simulink model "rmc_simulation"  (R2022b)
settings: Solver=ode45  StartTime=0.0  StopTime=50  FixedStep=0.01  RelTol=1e-3
settings Model: SimulationMode=accelerator  Creator=Adith JB  LastModifiedBy=Rohit
settings SolverCC: AlgebraicLoopSolver=TrustRegion
settings DataIOCC: LimitDataPoints=on  SaveFormat=Array  SignalLoggingSaveFormat=ModelDataLogs  ReturnWorkspaceOutputs=off
settings OptimizationCC: BlockReduction=off  BooleanDataType=off  ExpressionDepthLimit=2147483647  LifeSpan=inf
settings DebuggingCC: SaveWithParameterizedLinksMsg=none  UnderspecifiedInitializationDetection=Classic  MergeDetectMultiDrivingBlocksExec=none  SignalResolutionControl=TryResolveAllWithWarning  MultiTaskDSMMsg=warning  MultiTaskCondExecSysMsg=none  UnconnectedInputMsg=warning  UnconnectedOutputMsg=warning  UnconnectedLineMsg=warning  StateNameClashWarn=warning  SFUnexpectedBacktrackingDiag=warning  SFNoUnconditionalDefaultTransitionDiag=warning  SFExecutionAtInitializationDiag=none  SFMachineParentedDataDiag=warning  ArithmeticOperatorsInVariantConditions=warning
settings HardwareCC: ProdBitPerPointer=32  ProdBitPerSizeT=32  ProdBitPerPtrDiffT=32  ProdLargestAtomicFloat=None  ProdIntDivRoundTo=Undefined  ProdEndianess=Unspecified  ProdWordSize=32  ProdHWDeviceType=32-bit Generic  TargetUnknown=on
settings ModelReferenceCC: PropagateSignalLabelsOutOfModel=off
settings SFSimCC: SimUseLocalCustomCode=off  CustomCodeUndefinedFunction=UseInterfaceOnly
settings RTWCC: RTWUseLocalCustomCode=off
settings CodeAppCC: StateflowObjectComments=on
settings GRTTargetCC: TargetLangStandard=C89/C90 (ANSI)
settings ConfigComp: CovMetricSettings=dw  CovSaveCumulativeToWorkspaceVar=on  CovSaveSingleToWorkspaceVar=on  CovExternalEMLEnable=off

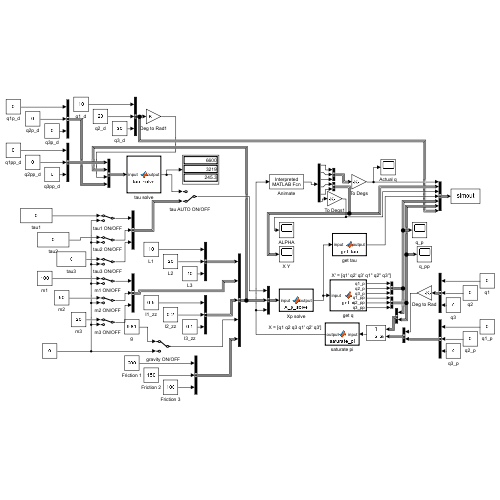
[thumbnail: Simulink's stored preview of the top-level diagram]
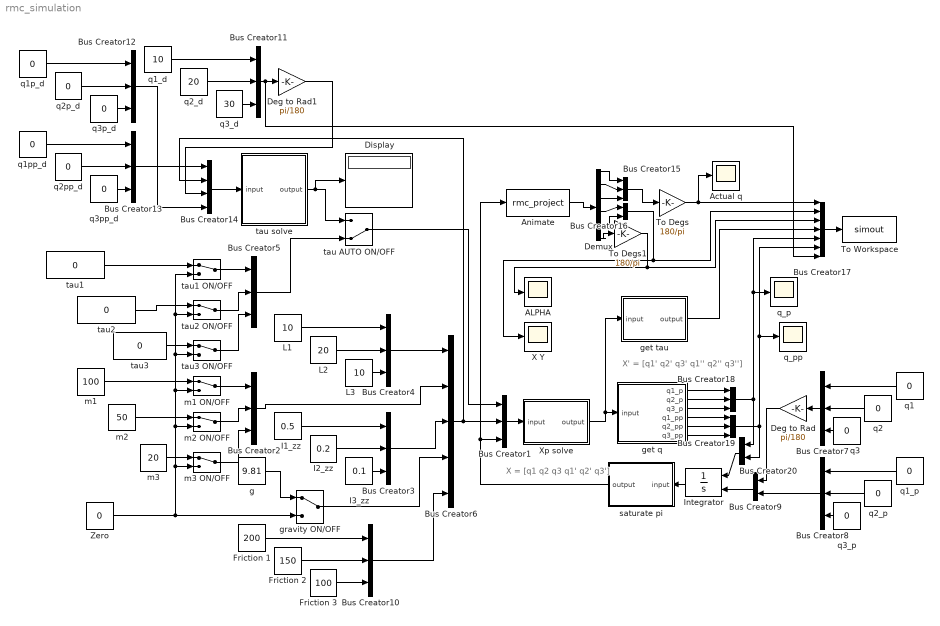
== system rmc_simulation ==
  note: X = [q1 q2 q3 q1' q2' q3']
  note: X' = [q1' q2' q3' q1'' q2'' q3'']
  ALPHA : Scope
  Actual q : Scope
  Animate : MATLABFcn  MATLABFcn=rmc_project  OutputDimensions=6  OutputSignalType=real
  Bus Creator{1..5,7..8,10..13,15,18..19} (14 alike) : BusCreator  Inputs=3
  Bus Creator14 : BusCreator  Inputs=4
  Bus Creator16 : BusCreator  Inputs=2
  Bus Creator17 : BusCreator  Inputs=7
  Bus Creator20 : BusCreator  Inputs=2
  Bus Creator6 : BusCreator  Inputs=5
  Bus Creator9 : BusCreator  Inputs=2
  Deg to Rad : Gain  Gain=pi/180
  Deg to Rad1 : Gain  Gain=pi/180
  Demux : Demux  Outputs=6
  Display : Display
  Friction 1 : Constant  Value=200
  Friction 2 : Constant  Value=150
  Friction 3 : Constant  Value=100
  I1_zz : Constant  Value=0.5
  I2_zz : Constant  Value=0.2
  I3_zz : Constant  Value=0.1
  Integrator : Integrator  InitialConditionSource=external
  L1 : Constant  Value=10
  L2 : Constant  Value=20
  L3 : Constant  Value=10
  To Degs : Gain  Gain=180/pi
  To Degs1 : Gain  Gain=180/pi
  To Workspace : ToWorkspace  VariableName=simout  SaveFormat=Structure With Time  SampleTime=-1
  X Y : Scope
  Xp solve : MATLAB Function  TreatAsAtomicUnit=on
  Zero : Constant  Value=0
  g : Constant  Value=9.81
  get q : MATLAB Function  TreatAsAtomicUnit=on
  get tau : MATLAB Function  TreatAsAtomicUnit=on
  gravity ON/OFF : ManualSwitch
  m1 : Constant  Value=100
  m1 ON/OFF : ManualSwitch
  m2 : Constant  Value=50
  m2 ON/OFF : ManualSwitch
  m3 : Constant  Value=20
  m3 ON/OFF : ManualSwitch
  q1 : Constant  Value=0
  q1_d : Constant  Value=10
  q1_p : Constant  Value=0
  q1p_d : Constant  Value=0
  q1pp_d : Constant  Value=0
  q2 : Constant  Value=0
  q2_d : Constant  Value=20
  q2_p : Constant  Value=0
  q2p_d : Constant  Value=0
  q2pp_d : Constant  Value=0
  q3 : Constant  Value=0
  q3_d : Constant  Value=30
  q3_p : Constant  Value=0
  q3p_d : Constant  Value=0
  q3pp_d : Constant  Value=0
  q_p : Scope
  q_pp : Scope
  saturate pi : MATLAB Function  TreatAsAtomicUnit=on
  tau AUTO ON/OFF : ManualSwitch  CurrentSetting=0
  tau solve : MATLAB Function  TreatAsAtomicUnit=on
  tau1 : Constant  Value=0
  tau1 ON/OFF : ManualSwitch
  tau2 : Constant  Value=0
  tau2 ON/OFF : ManualSwitch
  tau3 : Constant  Value=0
  tau3 ON/OFF : ManualSwitch
  wires:
  I1_zz/1 -> Bus Creator3/1
  I2_zz/1 -> Bus Creator3/2
  I3_zz/1 -> Bus Creator3/3
  L1/1 -> Bus Creator4/1
  L2/1 -> Bus Creator4/2
  L3/1 -> Bus Creator4/3
  Bus Creator4/1 -> Bus Creator6/1
  Bus Creator2/1 -> Bus Creator6/2
  Bus Creator3/1 -> Bus Creator6/3
  g/1 -> gravity ON/OFF/1
  gravity ON/OFF/1 -> Bus Creator6/4
  Bus Creator1/1 -> Xp solve/1(input)
  Bus Creator6/1 -> Bus Creator14/2, Bus Creator1/2
  To Degs/1 -> Bus Creator17/1, Actual q/1
  q1/1 -> Bus Creator7/1
  q2/1 -> Bus Creator7/2
  q3/1 -> Bus Creator7/3
  q1_p/1 -> Bus Creator8/1
  q2_p/1 -> Bus Creator8/2
  q3_p/1 -> Bus Creator8/3
  Bus Creator8/1 -> Bus Creator9/2
  Bus Creator7/1 -> Deg to Rad/1
  Deg to Rad/1 -> Bus Creator9/1
  Bus Creator9/1 -> Integrator/2
  m1/1 -> m1 ON/OFF/1
  m3 ON/OFF/1 -> Bus Creator2/3
  m3/1 -> m3 ON/OFF/1
  m1 ON/OFF/1 -> Bus Creator2/1
  m2 ON/OFF/1 -> Bus Creator2/2
  m2/1 -> m2 ON/OFF/1
  Integrator/1 -> saturate pi/1(input)
  Friction 3/1 -> Bus Creator10/3
  Friction 2/1 -> Bus Creator10/2
  Friction 1/1 -> Bus Creator10/1
  Bus Creator10/1 -> Bus Creator6/5
  tau1/1 -> tau1 ON/OFF/1
  tau2/1 -> tau2 ON/OFF/1
  Zero/1 -> gravity ON/OFF/2, tau1 ON/OFF/2, tau2 ON/OFF/2, tau3 ON/OFF/2, m1 ON/OFF/2, m2 ON/OFF/2, m3 ON/OFF/2
  tau3/1 -> tau3 ON/OFF/1
  tau3 ON/OFF/1 -> Bus Creator5/3
  tau2 ON/OFF/1 -> Bus Creator5/2
  tau1 ON/OFF/1 -> Bus Creator5/1
  tau solve/1(output) -> Display/1, tau AUTO ON/OFF/1
  Bus Creator5/1 -> tau AUTO ON/OFF/2
  tau AUTO ON/OFF/1 -> Bus Creator1/1
  q1_d/1 -> Bus Creator11/1
  q2_d/1 -> Bus Creator11/2
  q3_d/1 -> Bus Creator11/3
  q1p_d/1 -> Bus Creator12/1
  q2p_d/1 -> Bus Creator12/2
  q3p_d/1 -> Bus Creator12/3
  q1pp_d/1 -> Bus Creator13/1
  q2pp_d/1 -> Bus Creator13/2
  q3pp_d/1 -> Bus Creator13/3
  Bus Creator13/1 -> Bus Creator14/1
  Bus Creator11/1 -> Bus Creator17/7, Deg to Rad1/1
  Deg to Rad1/1 -> Bus Creator14/3
  Bus Creator12/1 -> Bus Creator14/4
  Bus Creator14/1 -> tau solve/1(input)
  saturate pi/1(output) -> Animate/1, Bus Creator1/3
  get tau/1(output) -> Bus Creator17/4
  Xp solve/1(output) -> get tau/1(input), get q/1(input)
  Animate/1 -> Demux/1
  Demux/1 -> Bus Creator15/1
  Demux/2 -> Bus Creator15/2
  Demux/3 -> Bus Creator15/3
  Bus Creator15/1 -> To Degs/1
  Bus Creator17/1 -> To Workspace/1
  get q/1(q1_p) -> Bus Creator18/1
  get q/2(q2_p) -> Bus Creator18/2
  get q/3(q3_p) -> Bus Creator18/3
  get q/4(q1_pp) -> Bus Creator19/1
  get q/5(q2_pp) -> Bus Creator19/2
  get q/6(q3_pp) -> Bus Creator19/3
  Bus Creator19/1 -> Bus Creator17/6, q_pp/1, Bus Creator20/2
  Bus Creator20/1 -> Integrator/1
  Bus Creator18/1 -> Bus Creator20/1, Bus Creator17/5, q_p/1
  Demux/4 -> Bus Creator16/1
  Demux/5 -> Bus Creator16/2
  Bus Creator16/1 -> X Y/1, Bus Creator17/2
  Demux/6 -> To Degs1/1
  To Degs1/1 -> Bus Creator17/3, ALPHA/1

== matlab function rmc_simulation/Xp solve ==
  data: input input; output output
function output  = X_p_solve(input)
    tau1 = input(1);
    tau2 = input(2);
    tau3 = input(3);
    L1 = input(4);
    L2 = input(5);
    L3 = input(6);
    m1 = input(7);
    m2 = input(8);
    m3 = input(9);
    I1_zz = input(10);
    I2_zz = input(11);
    I3_zz = input(12);
    g = input(13);
    D1 = input(14);
    D2 = input(15);
    D3 = input(16);
    q1 = input(17);
    q2 = input(18);
    q3 = input(19);
    q1_p = input(20);
    q2_p = input(21);
    q3_p = input(22);
    q1 = atan2(sin(q1),cos(q1));
    q2 = atan2(sin(q2),cos(q2));
    q3 = atan2(sin(q3),cos(q3));
    q1_pp = (2*(32*I2_zz*I3_zz*tau1 - 32*I2_zz*I3_zz*tau2 + 8*I3_zz*L2^2*m2*tau1 + 8*I2_zz*L3^2*m3*tau1 - 8*I3_zz*L2^2*m2*tau2 + 32*I3_zz*L2^2*m3*tau1 - 8*I2_zz*L3^2*m3*tau2 - 32*I3_zz*L2^2*m3*tau2 - 32*D1*I2_zz*I3_zz*q1_p + 32*D2*I2_zz*I3_zz*q2_p + 4*L2^2*L3^2*m3^2*tau1 - 4*L2^2*L3^2*m3^2*tau2 + 2*L2^2*L3^2*m2*m3*tau1 - 2*L2^2*L3^2*m2*m3*tau2 - 4*L2^2*L3^2*m3^2*tau1*cos(2*q3) + 4*L2^2*L3^2*m3^2*tau2*cos(2*q3) - 4*D1*L2^2*L3^2*m3^2*q1_p + 4*D2*L2^2*L3^2*m3^2*q2_p - 8*D1*I3_zz*L2^2*m2*q1_p - 8*D1*I2_zz*L3^2*m3*q1_p - 32*D1*I3_zz*L2^2*m3*q1_p + 8*D2*I3_zz*L2^2*m2*q2_p + 8*D2*I2_zz*L3^2*m3*q2_p + 32*D2*I3_zz*L2^2*m3*q2_p - 1120*I2_zz*I3_zz*L1*g*cos(q1) - 85*L1*L2^2*L3^2*g*m3^2*cos(q1) - 15*L1*L2^2*L3^2*g*m3^2*cos(q1 + 2*q2 + 2*q3) + 4*I2_zz*L1^2*L3^2*m3^2*q1_p^2*sin(2*q2 + 2*q3) + 4*I3_zz*L1*L2^3*m2^2*q1_p^2*sin(q2) + 4*I3_zz*L1*L2^3*m2^2*q2_p^2*sin(q2) + 32*I3_zz*L1*L2^3*m3^2*q1_p^2*sin(q2) + 32*I3_zz*L1*L2^3*m3^2*q2_p^2*sin(q2) + 15*L1*L2^2*L3^2*g*m3^2*cos(q1 + 2*q2) + 35*L1*L2^2*L3^2*g*m3^2*cos(q1 - 2*q3) + 50*L1*L2^2*L3^2*g*m3^2*cos(q1 + 2*q3) - 2*D1*L2^2*L3^2*m2*m3*q1_p + 2*D2*L2^2*L3^2*m2*m3*q2_p - 140*I3_zz*L1*L2^2*g*m2*cos(q1) - 240*I2_zz*L1*L3^2*g*m3*cos(q1) - 840*I3_zz*L1*L2^2*g*m3*cos(q1) + 40*I2_zz*L1*L3^2*g*m3*cos(q1 + 2*q2 + 2*q3) + 4*D1*L2^2*L3^2*m3^2*q1_p*cos(2*q3) - 4*D2*L2^2*L3^2*m3^2*q2_p*cos(2*q3) + 140*I3_zz*L1*L2^2*g*m2*cos(q1 + 2*q2) + 280*I3_zz*L1*L2^2*g*m3*cos(q1 + 2*q2) - 8*L1*L2^2*L3*m3^2*tau3*cos(q2 + q3) - 4*L1*L2*L3^2*m3^2*tau2*cos(q2) + 4*L1*L2*L3^2*m3^2*tau3*cos(q2) - 16*I2_zz*L1*L3*m3*tau3*cos(q2 + q3) + 4*I3_zz*L1^2*L2^2*m2^2*q1_p^2*sin(2*q2) + 16*I3_zz*L1^2*L2^2*m3^2*q1_p^2*sin(2*q2) + 4*L1*L2*L3^2*m3^2*tau2*cos(q2 + 2*q3) + 8*L1*L2^2*L3*m3^2*tau3*cos(q2 - q3) - 4*L1*L2*L3^2*m3^2*tau3*cos(q2 + 2*q3) + 4*I2_zz*L1*L3^3*m3^2*q1_p^2*sin(q2 + q3) + 4*I2_zz*L1*L3^3*m3^2*q2_p^2*sin(q2 + q3) + 4*I2_zz*L1*L3^3*m3^2*q3_p^2*sin(q2 + q3) - 16*I3_zz*L1*L2*m2*tau2*cos(q2) + 16*I3_zz*L1*L2*m2*tau3*cos(q2) - 32*I3_zz*L1*L2*m3*tau2*cos(q2) + 32*I3_zz*L1*L2*m3*tau3*cos(q2) + 8*I2_zz*L1*L3^3*m3^2*q1_p*q2_p*sin(q2 + q3) + 8*I2_zz*L1*L3^3*m3^2*q1_p*q3_p*sin(q2 + q3) + 8*I2_zz*L1*L3^3*m3^2*q2_p*q3_p*sin(q2 + q3) + 16*D3*I2_zz*L1*L3*m3*q3_p*cos(q2 + q3) - 35*L1*L2^2*L3^2*g*m2*m3*cos(q1) + L1*L2^2*L3^3*m2*m3^2*q1_p^2*sin(q2 - q3) + L1*L2^2*L3^3*m2*m3^2*q2_p^2*sin(q2 - q3) - L1*L2^3*L3^2*m2*m3^2*q1_p^2*sin(q2 + 2*q3) + L1*L2^2*L3^3*m2*m3^2*q3_p^2*sin(q2 - q3) - L1*L2^3*L3^2*m2*m3^2*q2_p^2*sin(q2 + 2*q3) - 4*D2*L1*L2*L3^2*m3^2*q2_p*cos(q2 + 2*q3) - 8*D3*L1*L2^2*L3*m3^2*q3_p*cos(q2 - q3) + 4*D3*L1*L2*L3^2*m3^2*q3_p*cos(q2 + 2*q3) + 24*I3_zz*L1*L2^3*m2*m3*q1_p^2*sin(q2) + 24*I3_zz*L1*L2^3*m2*m3*q2_p^2*sin(q2) + 8*I3_zz*L1*L2^3*m2^2*q1_p*q2_p*sin(q2) + 64*I3_zz*L1*L2^3*m3^2*q1_p*q2_p*sin(q2) + 16*D2*I3_zz*L1*L2*m2*q2_p*cos(q2) + 32*D2*I3_zz*L1*L2*m3*q2_p*cos(q2) - 16*D3*I3_zz*L1*L2*m2*q3_p*cos(q2) - 32*D3*I3_zz*L1*L2*m3*q3_p*cos(q2) + 8*I3_zz*L1*L2^2*L3*m3^2*q1_p^2*sin(q2 + q3) + 8*I3_zz*L1*L2^2*L3*m3^2*q2_p^2*sin(q2 + q3) + 8*I3_zz*L1*L2^2*L3*m3^2*q3_p^2*sin(q2 + q3) + 25*L1*L2^2*L3^2*g*m2*m3*cos(q1 + 2*q2) - 10*L1*L2^2*L3^2*g*m2*m3*cos(q1 + 2*q3) + 4*I2_zz*L1*L2*L3^2*m3^2*q1_p^2*sin(q2) + 4*I2_zz*L1*L2*L3^2*m3^2*q2_p^2*sin(q2) + 16*I2_zz*I3_zz*L1*L3*m3*q1_p^2*sin(q2 + q3) + 16*I2_zz*I3_zz*L1*L3*m3*q2_p^2*sin(q2 + q3) + 16*I2_zz*I3_zz*L1*L3*m3*q3_p^2*sin(q2 + q3) + 4*I2_zz*L1*L2*L3^2*m3^2*q1_p^2*sin(q2 + 2*q3) + 8*I3_zz*L1*L2^2*L3*m3^2*q1_p^2*sin(q2 - q3) + 4*I2_zz*L1*L2*L3^2*m3^2*q2_p^2*sin(q2 + 2*q3) + 8*I3_zz*L1*L2^2*L3*m3^2*q2_p^2*sin(q2 - q3) + 8*I3_zz*L1*L2^2*L3*m3^2*q3_p^2*sin(q2 - q3) + 16*I2_zz*I3_zz*L1*L2*m2*q1_p^2*sin(q2) + 16*I2_zz*I3_zz*L1*L2*m2*q2_p^2*sin(q2) + 32*I2_zz*I3_zz*L1*L2*m3*q1_p^2*sin(q2) + 32*I2_zz*I3_zz*L1*L2*m3*q2_p^2*sin(q2) + 2*L1^2*L2^2*L3^2*m2*m3^2*q1_p^2*sin(2*q2) + L1^2*L2^2*L3^2*m2^2*m3*q1_p^2*sin(2*q2) - 4*L1*L2*L3^2*m2*m3*tau2*cos(q2) + 4*L1*L2*L3^2*m2*m3*tau3*cos(q2) + 8*D3*L1*L2^2*L3*m3^2*q3_p*cos(q2 + q3) - L1^2*L2^2*L3^2*m2*m3^2*q1_p^2*sin(2*q2 + 2*q3) + 16*I3_zz*L1^2*L2^2*m2*m3*q1_p^2*sin(2*q2) + 3*L1*L2^3*L3^2*m2*m3^2*q1_p^2*sin(q2) + L1*L2^3*L3^2*m2^2*m3*q1_p^2*sin(q2) + 3*L1*L2^3*L3^2*m2*m3^2*q2_p^2*sin(q2) + L1*L2^3*L3^2*m2^2*m3*q2_p^2*sin(q2) + 4*L1*L2^2*L3*m2*m3*tau3*cos(q2 - q3) + 4*D2*L1*L2*L3^2*m3^2*q2_p*cos(q2) - 4*D3*L1*L2*L3^2*m3^2*q3_p*cos(q2) + 6*L1*L2^3*L3^2*m2*m3^2*q1_p*q2_p*sin(q2) + 2*L1*L2^3*L3^2*m2^2*m3*q1_p*q2_p*sin(q2) + 4*D2*L1*L2*L3^2*m2*m3*q2_p*cos(q2) - 4*D3*L1*L2*L3^2*m2*m3*q3_p*cos(q2) + 2*L1*L2^2*L3^3*m2*m3^2*q1_p*q2_p*sin(q2 - q3) + 2*L1*L2^2*L3^3*m2*m3^2*q1_p*q3_p*sin(q2 - q3) - 2*L1*L2^3*L3^2*m2*m3^2*q1_p*q2_p*sin(q2 + 2*q3) + 2*L1*L2^2*L3^3*m2*m3^2*q2_p*q3_p*sin(q2 - q3) - 4*D3*L1*L2^2*L3*m2*m3*q3_p*cos(q2 - q3) + 48*I3_zz*L1*L2^3*m2*m3*q1_p*q2_p*sin(q2) + 16*I3_zz*L1*L2^2*L3*m3^2*q1_p*q2_p*sin(q2 + q3) + 16*I3_zz*L1*L2^2*L3*m3^2*q1_p*q3_p*sin(q2 + q3) + 16*I3_zz*L1*L2^2*L3*m3^2*q2_p*q3_p*sin(q2 + q3) + 4*I2_zz*L1*L2*L3^2*m2*m3*q1_p^2*sin(q2) + 4*I2_zz*L1*L2*L3^2*m2*m3*q2_p^2*sin(q2) + 8*I2_zz*L1*L2*L3^2*m3^2*q1_p*q2_p*sin(q2) + 32*I2_zz*I3_zz*L1*L3*m3*q1_p*q2_p*sin(q2 + q3) + 32*I2_zz*I3_zz*L1*L3*m3*q1_p*q3_p*sin(q2 + q3) + 32*I2_zz*I3_zz*L1*L3*m3*q2_p*q3_p*sin(q2 + q3) + 4*I3_zz*L1*L2^2*L3*m2*m3*q1_p^2*sin(q2 - q3) + 4*I3_zz*L1*L2^2*L3*m2*m3*q2_p^2*sin(q2 - q3) + 4*I3_zz*L1*L2^2*L3*m2*m3*q3_p^2*sin(q2 - q3) + 8*I2_zz*L1*L2*L3^2*m3^2*q1_p*q2_p*sin(q2 + 2*q3) + 16*I3_zz*L1*L2^2*L3*m3^2*q1_p*q2_p*sin(q2 - q3) + 16*I3_zz*L1*L2^2*L3*m3^2*q1_p*q3_p*sin(q2 - q3) + 16*I3_zz*L1*L2^2*L3*m3^2*q2_p*q3_p*sin(q2 - q3) + 32*I2_zz*I3_zz*L1*L2*m2*q1_p*q2_p*sin(q2) + 64*I2_zz*I3_zz*L1*L2*m3*q1_p*q2_p*sin(q2) + 8*I2_zz*L1*L2*L3^2*m2*m3*q1_p*q2_p*sin(q2) + 8*I3_zz*L1*L2^2*L3*m2*m3*q1_p*q2_p*sin(q2 - q3) + 8*I3_zz*L1*L2^2*L3*m2*m3*q1_p*q3_p*sin(q2 - q3) + 8*I3_zz*L1*L2^2*L3*m2*m3*q2_p*q3_p*sin(q2 - q3)))/(64*I1_zz*I2_zz*I3_zz + 16*I2_zz*I3_zz*L1^2*m1 + 16*I1_zz*I3_zz*L2^2*m2 + 64*I2_zz*I3_zz*L1^2*m2 + 16*I1_zz*I2_zz*L3^2*m3 + 64*I1_zz*I3_zz*L2^2*m3 + 64*I2_zz*I3_zz*L1^2*m3 + 8*I3_zz*L1^2*L2^2*m2^2 + 8*I1_zz*L2^2*L3^2*m3^2 + 8*I2_zz*L1^2*L3^2*m3^2 + 32*I3_zz*L1^2*L2^2*m3^2 - 8*I2_zz*L1^2*L3^2*m3^2*cos(2*q2 + 2*q3) + 2*L1^2*L2^2*L3^2*m1*m3^2 + 6*L1^2*L2^2*L3^2*m2*m3^2 + 2*L1^2*L2^2*L3^2*m2^2*m3 + 4*I3_zz*L1^2*L2^2*m1*m2 + 4*I2_zz*L1^2*L3^2*m1*m3 + 16*I3_zz*L1^2*L2^2*m1*m3 + 4*I1_zz*L2^2*L3^2*m2*m3 + 16*I2_zz*L1^2*L3^2*m2*m3 + 48*I3_zz*L1^2*L2^2*m2*m3 - 8*I3_zz*L1^2*L2^2*m2^2*cos(2*q2) - 32*I3_zz*L1^2*L2^2*m3^2*cos(2*q2) - 8*I1_zz*L2^2*L3^2*m3^2*cos(2*q3) - 32*I3_zz*L1^2*L2^2*m2*m3*cos(2*q2) + L1^2*L2^2*L3^2*m1*m2*m3 - 2*L1^2*L2^2*L3^2*m1*m3^2*cos(2*q3) - 4*L1^2*L2^2*L3^2*m2*m3^2*cos(2*q2) - 2*L1^2*L2^2*L3^2*m2^2*m3*cos(2*q2) - 4*L1^2*L2^2*L3^2*m2*m3^2*cos(2*q3) + 2*L1^2*L2^2*L3^2*m2*m3^2*cos(2*q2 + 2*q3)); 
    q2_pp = -(2*(32*I2_zz*I3_zz*tau1 - 32*I1_zz*I3_zz*tau2 + 32*I1_zz*I3_zz*tau3 - 32*I2_zz*I3_zz*tau2 - 8*I3_zz*L1^2*m1*tau2 + 8*I3_zz*L1^2*m1*tau3 - 32*I3_zz*L1^2*m2*tau2 + 8*I3_zz*L2^2*m2*tau1 - 8*I1_zz*L3^2*m3*tau2 + 8*I2_zz*L3^2*m3*tau1 + 32*I3_zz*L1^2*m2*tau3 - 32*I3_zz*L1^2*m3*tau2 - 8*I3_zz*L2^2*m2*tau2 + 32*I3_zz*L2^2*m3*tau1 + 8*I1_zz*L3^2*m3*tau3 - 8*I2_zz*L3^2*m3*tau2 + 32*I3_zz*L1^2*m3*tau3 - 32*I3_zz*L2^2*m3*tau2 - 32*D1*I2_zz*I3_zz*q1_p + 32*D2*I1_zz*I3_zz*q2_p + 32*D2*I2_zz*I3_zz*q2_p - 32*D3*I1_zz*I3_zz*q3_p - 4*L1^2*L3^2*m3^2*tau2 + 4*L2^2*L3^2*m3^2*tau1 + 4*L1^2*L3^2*m3^2*tau3 - 4*L2^2*L3^2*m3^2*tau2 - 2*L1^2*L3^2*m1*m3*tau2 + 2*L1^2*L3^2*m1*m3*tau3 - 8*L1^2*L3^2*m2*m3*tau2 + 2*L2^2*L3^2*m2*m3*tau1 + 8*L1^2*L3^2*m2*m3*tau3 - 2*L2^2*L3^2*m2*m3*tau2 - 4*L2^2*L3^2*m3^2*tau1*cos(2*q3) + 4*L2^2*L3^2*m3^2*tau2*cos(2*q3) - 4*D1*L2^2*L3^2*m3^2*q1_p + 4*D2*L1^2*L3^2*m3^2*q2_p + 4*D2*L2^2*L3^2*m3^2*q2_p - 4*D3*L1^2*L3^2*m3^2*q3_p + 560*I1_zz*I3_zz*L2*g*cos(q1 + q2) + 4*L1^2*L3^2*m3^2*tau2*cos(2*q2 + 2*q3) - 4*L1^2*L3^2*m3^2*tau3*cos(2*q2 + 2*q3) - 8*D1*I3_zz*L2^2*m2*q1_p + 8*D2*I3_zz*L1^2*m1*q2_p - 8*D1*I2_zz*L3^2*m3*q1_p - 32*D1*I3_zz*L2^2*m3*q1_p + 32*D2*I3_zz*L1^2*m2*q2_p + 8*D2*I1_zz*L3^2*m3*q2_p + 32*D2*I3_zz*L1^2*m3*q2_p + 8*D2*I3_zz*L2^2*m2*q2_p - 8*D3*I3_zz*L1^2*m1*q3_p + 8*D2*I2_zz*L3^2*m3*q2_p + 32*D2*I3_zz*L2^2*m3*q2_p - 32*D3*I3_zz*L1^2*m2*q3_p - 8*D3*I1_zz*L3^2*m3*q3_p - 32*D3*I3_zz*L1^2*m3*q3_p - 1120*I2_zz*I3_zz*L1*g*cos(q1) - 85*L1*L2^2*L3^2*g*m3^2*cos(q1) + 35*L1^2*L2*L3^2*g*m3^2*cos(q1 - q2 - 2*q3) - 15*L1*L2^2*L3^2*g*m3^2*cos(q1 + 2*q2 + 2*q3) - 15*L1^2*L2*L3^2*g*m3^2*cos(q1 + 3*q2 + 2*q3) + 4*I2_zz*L1^2*L3^2*m3^2*q1_p^2*sin(2*q2 + 2*q3) + 140*I3_zz*L1^2*L2*g*m1*cos(q1 + q2) + 280*I3_zz*L1^2*L2*g*m2*cos(q1 + q2) + 100*I1_zz*L2*L3^2*g*m3*cos(q1 + q2) + 4*I3_zz*L1*L2^3*m2^2*q1_p^2*sin(q2) + 16*I3_zz*L1^3*L2*m2^2*q1_p^2*sin(q2) + 4*I3_zz*L1*L2^3*m2^2*q2_p^2*sin(q2) + 32*I3_zz*L1*L2^3*m3^2*q1_p^2*sin(q2) + 32*I3_zz*L1^3*L2*m3^2*q1_p^2*sin(q2) - 4*I1_zz*L2*L3^3*m3^2*q1_p^2*sin(q3) + 32*I3_zz*L1*L2^3*m3^2*q2_p^2*sin(q2) - 4*I1_zz*L2*L3^3*m3^2*q2_p^2*sin(q3) - 4*I1_zz*L2*L3^3*m3^2*q3_p^2*sin(q3) - 50*L1^2*L2*L3^2*g*m3^2*cos(q1 - q2) + 15*L1*L2^2*L3^2*g*m3^2*cos(q1 + 2*q2) + 35*L1*L2^2*L3^2*g*m3^2*cos(q1 - 2*q3) + 50*L1*L2^2*L3^2*g*m3^2*cos(q1 + 2*q3) - 2*D1*L2^2*L3^2*m2*m3*q1_p + 2*D2*L1^2*L3^2*m1*m3*q2_p + 8*D2*L1^2*L3^2*m2*m3*q2_p + 2*D2*L2^2*L3^2*m2*m3*q2_p - 2*D3*L1^2*L3^2*m1*m3*q3_p - 8*D3*L1^2*L3^2*m2*m3*q3_p - 140*I3_zz*L1*L2^2*g*m2*cos(q1) - 240*I2_zz*L1*L3^2*g*m3*cos(q1) - 840*I3_zz*L1*L2^2*g*m3*cos(q1) + 40*I2_zz*L1*L3^2*g*m3*cos(q1 + 2*q2 + 2*q3) + 4*D1*L2^2*L3^2*m3^2*q1_p*cos(2*q3) - 4*D2*L2^2*L3^2*m3^2*q2_p*cos(2*q3) - 280*I3_zz*L1^2*L2*g*m2*cos(q1 - q2) + 140*I3_zz*L1*L2^2*g*m2*cos(q1 + 2*q2) - 560*I3_zz*L1^2*L2*g*m3*cos(q1 - q2) + 280*I3_zz*L1*L2^2*g*m3*cos(q1 + 2*q2) - 8*L1*L2^2*L3*m3^2*tau3*cos(q2 + q3) - 4*D2*L1^2*L3^2*m3^2*q2_p*cos(2*q2 + 2*q3) + 4*D3*L1^2*L3^2*m3^2*q3_p*cos(2*q2 + 2*q3) + 50*L1^2*L2*L3^2*g*m3^2*cos(q1 + q2 + 2*q3) + 4*L1*L2*L3^2*m3^2*tau1*cos(q2) - 8*L1*L2*L3^2*m3^2*tau2*cos(q2) + 4*L1*L2*L3^2*m3^2*tau3*cos(q2) + 8*L1^2*L2*L3*m3^2*tau3*cos(q3) - 16*I2_zz*L1*L3*m3*tau3*cos(q2 + q3) - 20*L1^2*L2*L3^2*g*m3^2*cos(q1 + q2) + 8*I3_zz*L1^2*L2^2*m2^2*q1_p^2*sin(2*q2) + 4*I3_zz*L1^2*L2^2*m2^2*q2_p^2*sin(2*q2) + 32*I3_zz*L1^2*L2^2*m3^2*q1_p^2*sin(2*q2) - 4*I1_zz*L2^2*L3^2*m3^2*q1_p^2*sin(2*q3) + 16*I3_zz*L1^2*L2^2*m3^2*q2_p^2*sin(2*q2) - 4*I1_zz*L2^2*L3^2*m3^2*q2_p^2*sin(2*q3) - 4*L1*L2*L3^2*m3^2*tau1*cos(q2 + 2*q3) + 8*L1*L2*L3^2*m3^2*tau2*cos(q2 + 2*q3) + 8*L1*L2^2*L3*m3^2*tau3*cos(q2 - q3) - 4*L1*L2*L3^2*m3^2*tau3*cos(q2 + 2*q3) - 8*L1^2*L2*L3*m3^2*tau3*cos(2*q2 + q3) - 40*I1_zz*L2*L3^2*g*m3*cos(q1 + q2 + 2*q3) + 4*I2_zz*L1*L3^3*m3^2*q1_p^2*sin(q2 + q3) + 4*I2_zz*L1*L3^3*m3^2*q2_p^2*sin(q2 + q3) + 4*I2_zz*L1*L3^3*m3^2*q3_p^2*sin(q2 + q3) + 16*I3_zz*L1*L2*m2*tau1*cos(q2) - 32*I3_zz*L1*L2*m2*tau2*cos(q2) + 32*I3_zz*L1*L2*m3*tau1*cos(q2) + 16*I3_zz*L1*L2*m2*tau3*cos(q2) - 64*I3_zz*L1*L2*m3*tau2*cos(q2) + 32*I3_zz*L1*L2*m3*tau3*cos(q2) + 16*I1_zz*L2*L3*m3*tau3*cos(q3) + 8*I2_zz*L1*L3^3*m3^2*q1_p*q2_p*sin(q2 + q3) + 8*I2_zz*L1*L3^3*m3^2*q1_p*q3_p*sin(q2 + q3) + 8*I2_zz*L1*L3^3*m3^2*q2_p*q3_p*sin(q2 + q3) + 16*D3*I2_zz*L1*L3*m3*q3_p*cos(q2 + q3) - 35*L1*L2^2*L3^2*g*m2*m3*cos(q1) + 10*L1^2*L2*L3^2*g*m2*m3*cos(q1 + 3*q2 + 2*q3) + L1*L2^2*L3^3*m2*m3^2*q1_p^2*sin(q2 - q3) - L1^3*L2*L3^2*m1*m3^2*q1_p^2*sin(q2 + 2*q3) + L1*L2^2*L3^3*m2*m3^2*q2_p^2*sin(q2 - q3) - L1*L2^3*L3^2*m2*m3^2*q1_p^2*sin(q2 + 2*q3) + L1^2*L2*L3^3*m2*m3^2*q1_p^2*sin(2*q2 + q3) - 2*L1^3*L2*L3^2*m2*m3^2*q1_p^2*sin(q2 + 2*q3) + L1*L2^2*L3^3*m2*m3^2*q3_p^2*sin(q2 - q3) - L1*L2^3*L3^2*m2*m3^2*q2_p^2*sin(q2 + 2*q3) + L1^2*L2*L3^3*m2*m3^2*q2_p^2*sin(2*q2 + q3) + L1^2*L2*L3^3*m2*m3^2*q3_p^2*sin(2*q2 + q3) + 4*D1*L1*L2*L3^2*m3^2*q1_p*cos(q2 + 2*q3) - 8*D2*L1*L2*L3^2*m3^2*q2_p*cos(q2 + 2*q3) - 8*D3*L1*L2^2*L3*m3^2*q3_p*cos(q2 - q3) + 4*D3*L1*L2*L3^2*m3^2*q3_p*cos(q2 + 2*q3) + 8*D3*L1^2*L2*L3*m3^2*q3_p*cos(2*q2 + q3) + 4*I3_zz*L1^3*L2*m1*m2*q1_p^2*sin(q2) + 8*I3_zz*L1^3*L2*m1*m3*q1_p^2*sin(q2) + 24*I3_zz*L1*L2^3*m2*m3*q1_p^2*sin(q2) + 48*I3_zz*L1^3*L2*m2*m3*q1_p^2*sin(q2) + 24*I3_zz*L1*L2^3*m2*m3*q2_p^2*sin(q2) + 8*I3_zz*L1*L2^3*m2^2*q1_p*q2_p*sin(q2) + 64*I3_zz*L1*L2^3*m3^2*q1_p*q2_p*sin(q2) - 8*I1_zz*L2*L3^3*m3^2*q1_p*q2_p*sin(q3) - 8*I1_zz*L2*L3^3*m3^2*q1_p*q3_p*sin(q3) - 8*I1_zz*L2*L3^3*m3^2*q2_p*q3_p*sin(q3) - 16*D1*I3_zz*L1*L2*m2*q1_p*cos(q2) - 32*D1*I3_zz*L1*L2*m3*q1_p*cos(q2) + 32*D2*I3_zz*L1*L2*m2*q2_p*cos(q2) + 64*D2*I3_zz*L1*L2*m3*q2_p*cos(q2) - 16*D3*I3_zz*L1*L2*m2*q3_p*cos(q2) - 32*D3*I3_zz*L1*L2*m3*q3_p*cos(q2) - 16*D3*I1_zz*L2*L3*m3*q3_p*cos(q3) + 8*I3_zz*L1*L2^2*L3*m3^2*q1_p^2*sin(q2 + q3) + 8*I3_zz*L1*L2^2*L3*m3^2*q2_p^2*sin(q2 + q3) + 8*I3_zz*L1*L2^2*L3*m3^2*q3_p^2*sin(q2 + q3) - 60*L1^2*L2*L3^2*g*m2*m3*cos(q1 - q2) + 25*L1*L2^2*L3^2*g*m2*m3*cos(q1 + 2*q2) - 10*L1*L2^2*L3^2*g*m2*m3*cos(q1 + 2*q3) + 4*I1_zz*L1*L2*L3^2*m3^2*q1_p^2*sin(q2) + 4*I2_zz*L1*L2*L3^2*m3^2*q1_p^2*sin(q2) + 4*I2_zz*L1*L2*L3^2*m3^2*q2_p^2*sin(q2) - 8*I3_zz*L1^2*L2*L3*m3^2*q1_p^2*sin(q3) - 8*I3_zz*L1^2*L2*L3*m3^2*q2_p^2*sin(q3) - 8*I3_zz*L1^2*L2*L3*m3^2*q3_p^2*sin(q3) + 16*I2_zz*I3_zz*L1*L3*m3*q1_p^2*sin(q2 + q3) + 16*I2_zz*I3_zz*L1*L3*m3*q2_p^2*sin(q2 + q3) + 16*I2_zz*I3_zz*L1*L3*m3*q3_p^2*sin(q2 + q3) - 4*I1_zz*L1*L2*L3^2*m3^2*q1_p^2*sin(q2 + 2*q3) + 4*I2_zz*L1*L2*L3^2*m3^2*q1_p^2*sin(q2 + 2*q3) + 8*I3_zz*L1*L2^2*L3*m3^2*q1_p^2*sin(q2 - q3) + 4*I2_zz*L1*L2*L3^2*m3^2*q2_p^2*sin(q2 + 2*q3) + 8*I3_zz*L1*L2^2*L3*m3^2*q2_p^2*sin(q2 - q3) + 8*I3_zz*L1^2*L2*L3*m3^2*q1_p^2*sin(2*q2 + q3) + 8*I3_zz*L1*L2^2*L3*m3^2*q3_p^2*sin(q2 - q3) + 8*I3_zz*L1^2*L2*L3*m3^2*q2_p^2*sin(2*q2 + q3) + 8*I3_zz*L1^2*L2*L3*m3^2*q3_p^2*sin(2*q2 + q3) + 16*I1_zz*I3_zz*L1*L2*m2*q1_p^2*sin(q2) + 32*I1_zz*I3_zz*L1*L2*m3*q1_p^2*sin(q2) + 16*I2_zz*I3_zz*L1*L2*m2*q1_p^2*sin(q2) + 16*I2_zz*I3_zz*L1*L2*m2*q2_p^2*sin(q2) + 32*I2_zz*I3_zz*L1*L2*m3*q1_p^2*sin(q2) + 32*I2_zz*I3_zz*L1*L2*m3*q2_p^2*sin(q2) - 16*I1_zz*I3_zz*L2*L3*m3*q1_p^2*sin(q3) - 16*I1_zz*I3_zz*L2*L3*m3*q2_p^2*sin(q3) - 16*I1_zz*I3_zz*L2*L3*m3*q3_p^2*sin(q3) - L1^2*L2^2*L3^2*m1*m3^2*q1_p^2*sin(2*q3) + 4*L1^2*L2^2*L3^2*m2*m3^2*q1_p^2*sin(2*q2) + 2*L1^2*L2^2*L3^2*m2^2*m3*q1_p^2*sin(2*q2) - L1^2*L2^2*L3^2*m1*m3^2*q2_p^2*sin(2*q3) - 2*L1^2*L2^2*L3^2*m2*m3^2*q1_p^2*sin(2*q3) + 2*L1^2*L2^2*L3^2*m2*m3^2*q2_p^2*sin(2*q2) + L1^2*L2^2*L3^2*m2^2*m3*q2_p^2*sin(2*q2) - 2*L1^2*L2^2*L3^2*m2*m3^2*q2_p^2*sin(2*q3) - 10*L1^2*L2*L3^2*g*m1*m3*cos(q1 + q2 + 2*q3) - 30*L1^2*L2*L3^2*g*m2*m3*cos(q1 + q2 + 2*q3) + 4*L1*L2*L3^2*m2*m3*tau1*cos(q2) - 8*L1*L2*L3^2*m2*m3*tau2*cos(q2) + 4*L1*L2*L3^2*m2*m3*tau3*cos(q2) + 4*L1^2*L2*L3*m1*m3*tau3*cos(q3) + 12*L1^2*L2*L3*m2*m3*tau3*cos(q3) + 8*D3*L1*L2^2*L3*m3^2*q3_p*cos(q2 + q3) - L1^2*L2^2*L3^2*m2*m3^2*q1_p^2*sin(2*q2 + 2*q3) + 25*L1^2*L2*L3^2*g*m1*m3*cos(q1 + q2) + 40*L1^2*L2*L3^2*g*m2*m3*cos(q1 + q2) + 32*I3_zz*L1^2*L2^2*m2*m3*q1_p^2*sin(2*q2) + 16*I3_zz*L1^2*L2^2*m2*m3*q2_p^2*sin(2*q2) + L1^3*L2*L3^2*m1*m3^2*q1_p^2*sin(q2) + 3*L1*L2^3*L3^2*m2*m3^2*q1_p^2*sin(q2) + L1*L2^3*L3^2*m2^2*m3*q1_p^2*sin(q2) - L1^2*L2*L3^3*m1*m3^2*q1_p^2*sin(q3) + 6*L1^3*L2*L3^2*m2*m3^2*q1_p^2*sin(q2) + 4*L1^3*L2*L3^2*m2^2*m3*q1_p^2*sin(q2) + 3*L1*L2^3*L3^2*m2*m3^2*q2_p^2*sin(q2) + L1*L2^3*L3^2*m2^2*m3*q2_p^2*sin(q2) - L1^2*L2*L3^3*m1*m3^2*q2_p^2*sin(q3) - 3*L1^2*L2*L3^3*m2*m3^2*q1_p^2*sin(q3) - L1^2*L2*L3^3*m1*m3^2*q3_p^2*sin(q3) - 3*L1^2*L2*L3^3*m2*m3^2*q2_p^2*sin(q3) - 3*L1^2*L2*L3^3*m2*m3^2*q3_p^2*sin(q3) + 8*I3_zz*L1^2*L2^2*m2^2*q1_p*q2_p*sin(2*q2) + 32*I3_zz*L1^2*L2^2*m3^2*q1_p*q2_p*sin(2*q2) - 8*I1_zz*L2^2*L3^2*m3^2*q1_p*q2_p*sin(2*q3) + 4*L1*L2^2*L3*m2*m3*tau3*cos(q2 - q3) - 4*L1^2*L2*L3*m2*m3*tau3*cos(2*q2 + q3) - 4*D1*L1*L2*L3^2*m3^2*q1_p*cos(q2) + 8*D2*L1*L2*L3^2*m3^2*q2_p*cos(q2) - 4*D3*L1*L2*L3^2*m3^2*q3_p*cos(q2) - 8*D3*L1^2*L2*L3*m3^2*q3_p*cos(q3) + 6*L1*L2^3*L3^2*m2*m3^2*q1_p*q2_p*sin(q2) + 2*L1*L2^3*L3^2*m2^2*m3*q1_p*q2_p*sin(q2) - 2*L1^2*L2*L3^3*m1*m3^2*q1_p*q2_p*sin(q3) - 2*L1^2*L2*L3^3*m1*m3^2*q1_p*q3_p*sin(q3) - 6*L1^2*L2*L3^3*m2*m3^2*q1_p*q2_p*sin(q3) - 2*L1^2*L2*L3^3*m1*m3^2*q2_p*q3_p*sin(q3) - 6*L1^2*L2*L3^3*m2*m3^2*q1_p*q3_p*sin(q3) - 6*L1^2*L2*L3^3*m2*m3^2*q2_p*q3_p*sin(q3) - 4*D1*L1*L2*L3^2*m2*m3*q1_p*cos(q2) + 8*D2*L1*L2*L3^2*m2*m3*q2_p*cos(q2) - 4*D3*L1*L2*L3^2*m2*m3*q3_p*cos(q2) - 4*D3*L1^2*L2*L3*m1*m3*q3_p*cos(q3) - 12*D3*L1^2*L2*L3*m2*m3*q3_p*cos(q3) + 2*L1*L2^2*L3^3*m2*m3^2*q1_p*q2_p*sin(q2 - q3) + 2*L1*L2^2*L3^3*m2*m3^2*q1_p*q3_p*sin(q2 - q3) - 2*L1*L2^3*L3^2*m2*m3^2*q1_p*q2_p*sin(q2 + 2*q3) + 2*L1^2*L2*L3^3*m2*m3^2*q1_p*q2_p*sin(2*q2 + q3) + 2*L1*L2^2*L3^3*m2*m3^2*q2_p*q3_p*sin(q2 - q3) + 2*L1^2*L2*L3^3*m2*m3^2*q1_p*q3_p*sin(2*q2 + q3) + 2*L1^2*L2*L3^3*m2*m3^2*q2_p*q3_p*sin(2*q2 + q3) - 4*D3*L1*L2^2*L3*m2*m3*q3_p*cos(q2 - q3) + 4*D3*L1^2*L2*L3*m2*m3*q3_p*cos(2*q2 + q3) + 48*I3_zz*L1*L2^3*m2*m3*q1_p*q2_p*sin(q2) + 16*I3_zz*L1*L2^2*L3*m3^2*q1_p*q2_p*sin(q2 + q3) + 16*I3_zz*L1*L2^2*L3*m3^2*q1_p*q3_p*sin(q2 + q3) + 16*I3_zz*L1*L2^2*L3*m3^2*q2_p*q3_p*sin(q2 + q3) + 4*I1_zz*L1*L2*L3^2*m2*m3*q1_p^2*sin(q2) + 4*I2_zz*L1*L2*L3^2*m2*m3*q1_p^2*sin(q2) + 4*I2_zz*L1*L2*L3^2*m2*m3*q2_p^2*sin(q2) - 4*I3_zz*L1^2*L2*L3*m1*m3*q1_p^2*sin(q3) - 4*I3_zz*L1^2*L2*L3*m1*m3*q2_p^2*sin(q3) - 12*I3_zz*L1^2*L2*L3*m2*m3*q1_p^2*sin(q3) - 4*I3_zz*L1^2*L2*L3*m1*m3*q3_p^2*sin(q3) - 12*I3_zz*L1^2*L2*L3*m2*m3*q2_p^2*sin(q3) - 12*I3_zz*L1^2*L2*L3*m2*m3*q3_p^2*sin(q3) + 8*I2_zz*L1*L2*L3^2*m3^2*q1_p*q2_p*sin(q2) - 16*I3_zz*L1^2*L2*L3*m3^2*q1_p*q2_p*sin(q3) - 16*I3_zz*L1^2*L2*L3*m3^2*q1_p*q3_p*sin(q3) - 16*I3_zz*L1^2*L2*L3*m3^2*q2_p*q3_p*sin(q3) + 32*I2_zz*I3_zz*L1*L3*m3*q1_p*q2_p*sin(q2 + q3) + 32*I2_zz*I3_zz*L1*L3*m3*q1_p*q3_p*sin(q2 + q3) + 32*I2_zz*I3_zz*L1*L3*m3*q2_p*q3_p*sin(q2 + q3) + 4*I3_zz*L1*L2^2*L3*m2*m3*q1_p^2*sin(q2 - q3) + 4*I3_zz*L1*L2^2*L3*m2*m3*q2_p^2*sin(q2 - q3) + 4*I3_zz*L1^2*L2*L3*m2*m3*q1_p^2*sin(2*q2 + q3) + 4*I3_zz*L1*L2^2*L3*m2*m3*q3_p^2*sin(q2 - q3) + 4*I3_zz*L1^2*L2*L3*m2*m3*q2_p^2*sin(2*q2 + q3) + 4*I3_zz*L1^2*L2*L3*m2*m3*q3_p^2*sin(2*q2 + q3) + 8*I2_zz*L1*L2*L3^2*m3^2*q1_p*q2_p*sin(q2 + 2*q3) + 16*I3_zz*L1*L2^2*L3*m3^2*q1_p*q2_p*sin(q2 - q3) + 16*I3_zz*L1*L2^2*L3*m3^2*q1_p*q3_p*sin(q2 - q3) + 16*I3_zz*L1^2*L2*L3*m3^2*q1_p*q2_p*sin(2*q2 + q3) + 16*I3_zz*L1*L2^2*L3*m3^2*q2_p*q3_p*sin(q2 - q3) + 16*I3_zz*L1^2*L2*L3*m3^2*q1_p*q3_p*sin(2*q2 + q3) + 16*I3_zz*L1^2*L2*L3*m3^2*q2_p*q3_p*sin(2*q2 + q3) + 32*I2_zz*I3_zz*L1*L2*m2*q1_p*q2_p*sin(q2) + 64*I2_zz*I3_zz*L1*L2*m3*q1_p*q2_p*sin(q2) - 32*I1_zz*I3_zz*L2*L3*m3*q1_p*q2_p*sin(q3) - 32*I1_zz*I3_zz*L2*L3*m3*q1_p*q3_p*sin(q3) - 32*I1_zz*I3_zz*L2*L3*m3*q2_p*q3_p*sin(q3) - 2*L1^2*L2^2*L3^2*m1*m3^2*q1_p*q2_p*sin(2*q3) + 4*L1^2*L2^2*L3^2*m2*m3^2*q1_p*q2_p*sin(2*q2) + 2*L1^2*L2^2*L3^2*m2^2*m3*q1_p*q2_p*sin(2*q2) - 4*L1^2*L2^2*L3^2*m2*m3^2*q1_p*q2_p*sin(2*q3) + L1^3*L2*L3^2*m1*m2*m3*q1_p^2*sin(q2) + 32*I3_zz*L1^2*L2^2*m2*m3*q1_p*q2_p*sin(2*q2) + 8*I2_zz*L1*L2*L3^2*m2*m3*q1_p*q2_p*sin(q2) - 8*I3_zz*L1^2*L2*L3*m1*m3*q1_p*q2_p*sin(q3) - 8*I3_zz*L1^2*L2*L3*m1*m3*q1_p*q3_p*sin(q3) - 24*I3_zz*L1^2*L2*L3*m2*m3*q1_p*q2_p*sin(q3) - 8*I3_zz*L1^2*L2*L3*m1*m3*q2_p*q3_p*sin(q3) - 24*I3_zz*L1^2*L2*L3*m2*m3*q1_p*q3_p*sin(q3) - 24*I3_zz*L1^2*L2*L3*m2*m3*q2_p*q3_p*sin(q3) + 8*I3_zz*L1*L2^2*L3*m2*m3*q1_p*q2_p*sin(q2 - q3) + 8*I3_zz*L1*L2^2*L3*m2*m3*q1_p*q3_p*sin(q2 - q3) + 8*I3_zz*L1^2*L2*L3*m2*m3*q1_p*q2_p*sin(2*q2 + q3) + 8*I3_zz*L1*L2^2*L3*m2*m3*q2_p*q3_p*sin(q2 - q3) + 8*I3_zz*L1^2*L2*L3*m2*m3*q1_p*q3_p*sin(2*q2 + q3) + 8*I3_zz*L1^2*L2*L3*m2*m3*q2_p*q3_p*sin(2*q2 + q3)))/(64*I1_zz*I2_zz*I3_zz + 16*I2_zz*I3_zz*L1^2*m1 + 16*I1_zz*I3_zz*L2^2*m2 + 64*I2_zz*I3_zz*L1^2*m2 + 16*I1_zz*I2_zz*L3^2*m3 + 64*I1_zz*I3_zz*L2^2*m3 + 64*I2_zz*I3_zz*L1^2*m3 + 8*I3_zz*L1^2*L2^2*m2^2 + 8*I1_zz*L2^2*L3^2*m3^2 + 8*I2_zz*L1^2*L3^2*m3^2 + 32*I3_zz*L1^2*L2^2*m3^2 - 8*I2_zz*L1^2*L3^2*m3^2*cos(2*q2 + 2*q3) + 2*L1^2*L2^2*L3^2*m1*m3^2 + 6*L1^2*L2^2*L3^2*m2*m3^2 + 2*L1^2*L2^2*L3^2*m2^2*m3 + 4*I3_zz*L1^2*L2^2*m1*m2 + 4*I2_zz*L1^2*L3^2*m1*m3 + 16*I3_zz*L1^2*L2^2*m1*m3 + 4*I1_zz*L2^2*L3^2*m2*m3 + 16*I2_zz*L1^2*L3^2*m2*m3 + 48*I3_zz*L1^2*L2^2*m2*m3 - 8*I3_zz*L1^2*L2^2*m2^2*cos(2*q2) - 32*I3_zz*L1^2*L2^2*m3^2*cos(2*q2) - 8*I1_zz*L2^2*L3^2*m3^2*cos(2*q3) - 32*I3_zz*L1^2*L2^2*m2*m3*cos(2*q2) + L1^2*L2^2*L3^2*m1*m2*m3 - 2*L1^2*L2^2*L3^2*m1*m3^2*cos(2*q3) - 4*L1^2*L2^2*L3^2*m2*m3^2*cos(2*q2) - 2*L1^2*L2^2*L3^2*m2^2*m3*cos(2*q2) - 4*L1^2*L2^2*L3^2*m2*m3^2*cos(2*q3) + 2*L1^2*L2^2*L3^2*m2*m3^2*cos(2*q2 + 2*q3));
    q3_pp = -(2*(32*I1_zz*I3_zz*tau2 - 32*I1_zz*I2_zz*tau3 - 32*I1_zz*I3_zz*tau3 - 8*I2_zz*L1^2*m1*tau3 + 8*I3_zz*L1^2*m1*tau2 - 8*I1_zz*L2^2*m2*tau3 - 32*I2_zz*L1^2*m2*tau3 - 8*I3_zz*L1^2*m1*tau3 + 32*I3_zz*L1^2*m2*tau2 - 32*I1_zz*L2^2*m3*tau3 + 8*I1_zz*L3^2*m3*tau2 - 32*I2_zz*L1^2*m3*tau3 - 32*I3_zz*L1^2*m2*tau3 + 32*I3_zz*L1^2*m3*tau2 - 8*I1_zz*L3^2*m3*tau3 - 32*I3_zz*L1^2*m3*tau3 - 32*D2*I1_zz*I3_zz*q2_p + 32*D3*I1_zz*I2_zz*q3_p + 32*D3*I1_zz*I3_zz*q3_p - 4*L1^2*L2^2*m2^2*tau3 - 16*L1^2*L2^2*m3^2*tau3 + 4*L1^2*L3^2*m3^2*tau2 - 4*L1^2*L3^2*m3^2*tau3 - 2*L1^2*L2^2*m1*m2*tau3 - 8*L1^2*L2^2*m1*m3*tau3 + 2*L1^2*L3^2*m1*m3*tau2 - 24*L1^2*L2^2*m2*m3*tau3 - 2*L1^2*L3^2*m1*m3*tau3 + 8*L1^2*L3^2*m2*m3*tau2 - 8*L1^2*L3^2*m2*m3*tau3 + 4*L1^2*L2^2*m2^2*tau3*cos(2*q2) + 16*L1^2*L2^2*m3^2*tau3*cos(2*q2) - 4*D2*L1^2*L3^2*m3^2*q2_p + 4*D3*L1^2*L2^2*m2^2*q3_p + 16*D3*L1^2*L2^2*m3^2*q3_p + 4*D3*L1^2*L3^2*m3^2*q3_p - 560*I1_zz*I3_zz*L2*g*cos(q1 + q2) - 4*L1^2*L3^2*m3^2*tau2*cos(2*q2 + 2*q3) + 4*L1^2*L3^2*m3^2*tau3*cos(2*q2 + 2*q3) - 8*D2*I3_zz*L1^2*m1*q2_p - 32*D2*I3_zz*L1^2*m2*q2_p + 8*D3*I2_zz*L1^2*m1*q3_p - 8*D2*I1_zz*L3^2*m3*q2_p - 32*D2*I3_zz*L1^2*m3*q2_p + 8*D3*I1_zz*L2^2*m2*q3_p + 32*D3*I2_zz*L1^2*m2*q3_p + 8*D3*I3_zz*L1^2*m1*q3_p + 32*D3*I1_zz*L2^2*m3*q3_p + 32*D3*I2_zz*L1^2*m3*q3_p + 32*D3*I3_zz*L1^2*m2*q3_p + 8*D3*I1_zz*L3^2*m3*q3_p + 32*D3*I3_zz*L1^2*m3*q3_p + 160*I1_zz*I2_zz*L3*g*cos(q1 + q2 + q3) - 70*L1^2*L2^2*L3*g*m3^2*cos(q1 - q2 - q3) - 35*L1^2*L2*L3^2*g*m3^2*cos(q1 - q2 - 2*q3) + 15*L1^2*L2*L3^2*g*m3^2*cos(q1 + 3*q2 + 2*q3) + 4*I2_zz*L1^2*L3^2*m3^2*q1_p^2*sin(2*q2 + 2*q3) + 4*I2_zz*L1^2*L3^2*m3^2*q2_p^2*sin(2*q2 + 2*q3) + 4*I2_zz*L1^2*L3^2*m3^2*q3_p^2*sin(2*q2 + 2*q3) - 140*I3_zz*L1^2*L2*g*m1*cos(q1 + q2) - 280*I3_zz*L1^2*L2*g*m2*cos(q1 + q2) - 100*I1_zz*L2*L3^2*g*m3*cos(q1 + q2) - 16*I3_zz*L1^3*L2*m2^2*q1_p^2*sin(q2) - 32*I3_zz*L1^3*L2*m3^2*q1_p^2*sin(q2) + 4*I1_zz*L2*L3^3*m3^2*q1_p^2*sin(q3) + 16*I1_zz*L2^3*L3*m3^2*q1_p^2*sin(q3) + 4*I1_zz*L2*L3^3*m3^2*q2_p^2*sin(q3) + 16*I1_zz*L2^3*L3*m3^2*q2_p^2*sin(q3) + 4*I1_zz*L2*L3^3*m3^2*q3_p^2*sin(q3) + 16*L1^2*L2^2*m2*m3*tau3*cos(2*q2) + 50*L1^2*L2*L3^2*g*m3^2*cos(q1 - q2) - 2*D2*L1^2*L3^2*m1*m3*q2_p + 2*D3*L1^2*L2^2*m1*m2*q3_p - 8*D2*L1^2*L3^2*m2*m3*q2_p + 8*D3*L1^2*L2^2*m1*m3*q3_p + 24*D3*L1^2*L2^2*m2*m3*q3_p + 2*D3*L1^2*L3^2*m1*m3*q3_p + 8*D3*L1^2*L3^2*m2*m3*q3_p - 280*I2_zz*L1^2*L3*g*m3*cos(q1 - q2 - q3) + 20*L1^2*L2^2*L3*g*m2^2*cos(q1 + q2 + q3) - 130*L1^2*L2^2*L3*g*m3^2*cos(q1 + q2 + q3) - 4*D3*L1^2*L2^2*m2^2*q3_p*cos(2*q2) - 16*D3*L1^2*L2^2*m3^2*q3_p*cos(2*q2) + 280*I3_zz*L1^2*L2*g*m2*cos(q1 - q2) + 560*I3_zz*L1^2*L2*g*m3*cos(q1 - q2) + 8*L1*L2^2*L3*m3^2*tau1*cos(q2 + q3) - 8*L1*L2^2*L3*m3^2*tau2*cos(q2 + q3) + 40*I2_zz*L1^2*L3*g*m1*cos(q1 + q2 + q3) + 40*I1_zz*L2^2*L3*g*m2*cos(q1 + q2 + q3) + 160*I2_zz*L1^2*L3*g*m2*cos(q1 + q2 + q3) + 20*I1_zz*L2^2*L3*g*m3*cos(q1 + q2 + q3) - 120*I2_zz*L1^2*L3*g*m3*cos(q1 + q2 + q3) + 4*D2*L1^2*L3^2*m3^2*q2_p*cos(2*q2 + 2*q3) - 4*D3*L1^2*L3^2*m3^2*q3_p*cos(2*q2 + 2*q3) - 10*L1^2*L2^2*L3*g*m2^2*cos(q1 - q2 + q3) + 70*L1^2*L2^2*L3*g*m3^2*cos(q1 + q2 - q3) + 100*L1^2*L2^2*L3*g*m3^2*cos(q1 - q2 + q3) - 50*L1^2*L2*L3^2*g*m3^2*cos(q1 + q2 + 2*q3) - 10*L1^2*L2^2*L3*g*m2^2*cos(q1 + 3*q2 + q3) + 30*L1^2*L2^2*L3*g*m3^2*cos(q1 + 3*q2 + q3) - 4*L1*L2*L3^2*m3^2*tau1*cos(q2) + 4*L1*L2*L3^2*m3^2*tau2*cos(q2) + 8*L1^2*L2*L3*m3^2*tau2*cos(q3) - 16*L1^2*L2*L3*m3^2*tau3*cos(q3) + 16*I2_zz*L1*L3*m3*tau1*cos(q2 + q3) - 16*I2_zz*L1*L3*m3*tau2*cos(q2 + q3) + 20*L1^2*L2*L3^2*g*m3^2*cos(q1 + q2) - 4*I3_zz*L1^2*L2^2*m2^2*q1_p^2*sin(2*q2) - 4*I3_zz*L1^2*L2^2*m2^2*q2_p^2*sin(2*q2) - 16*I3_zz*L1^2*L2^2*m3^2*q1_p^2*sin(2*q2) + 8*I1_zz*L2^2*L3^2*m3^2*q1_p^2*sin(2*q3) - 16*I3_zz*L1^2*L2^2*m3^2*q2_p^2*sin(2*q2) + 8*I1_zz*L2^2*L3^2*m3^2*q2_p^2*sin(2*q3) + 4*I1_zz*L2^2*L3^2*m3^2*q3_p^2*sin(2*q3) - 8*L1*L2^2*L3*m3^2*tau1*cos(q2 - q3) + 4*L1*L2*L3^2*m3^2*tau1*cos(q2 + 2*q3) + 8*L1*L2^2*L3*m3^2*tau2*cos(q2 - q3) - 4*L1*L2*L3^2*m3^2*tau2*cos(q2 + 2*q3) - 8*L1^2*L2*L3*m3^2*tau2*cos(2*q2 + q3) + 16*L1^2*L2*L3*m3^2*tau3*cos(2*q2 + q3) - 140*I1_zz*L2^2*L3*g*m3*cos(q1 + q2 - q3) + 40*I1_zz*L2*L3^2*g*m3*cos(q1 + q2 + 2*q3) + 16*I2_zz*L1^3*L3*m3^2*q1_p^2*sin(q2 + q3) - 16*I3_zz*L1*L2*m2*tau1*cos(q2) + 16*I3_zz*L1*L2*m2*tau2*cos(q2) - 32*I3_zz*L1*L2*m3*tau1*cos(q2) + 32*I3_zz*L1*L2*m3*tau2*cos(q2) + 16*I1_zz*L2*L3*m3*tau2*cos(q3) - 32*I1_zz*L2*L3*m3*tau3*cos(q3) - 16*D1*I2_zz*L1*L3*m3*q1_p*cos(q2 + q3) + 16*D2*I2_zz*L1*L3*m3*q2_p*cos(q2 + q3) + 35*L1^2*L2^2*L3*g*m2*m3*cos(q1 - q2 - q3) - 10*L1^2*L2*L3^2*g*m2*m3*cos(q1 + 3*q2 + 2*q3) - 2*L1^3*L2^2*L3*m1*m3^2*q1_p^2*sin(q2 - q3) + L1^3*L2*L3^2*m1*m3^2*q1_p^2*sin(q2 + 2*q3) - 4*L1^3*L2^2*L3*m2*m3^2*q1_p^2*sin(q2 - q3) - 2*L1^3*L2^2*L3*m2^2*m3*q1_p^2*sin(q2 - q3) - L1^2*L2*L3^3*m2*m3^2*q1_p^2*sin(2*q2 + q3) - 2*L1^2*L2^3*L3*m2*m3^2*q1_p^2*sin(2*q2 + q3) - L1^2*L2^3*L3*m2^2*m3*q1_p^2*sin(2*q2 + q3) + 2*L1^3*L2*L3^2*m2*m3^2*q1_p^2*sin(q2 + 2*q3) - L1^2*L2*L3^3*m2*m3^2*q2_p^2*sin(2*q2 + q3) - 2*L1^2*L2^3*L3*m2*m3^2*q2_p^2*sin(2*q2 + q3) - L1^2*L2^3*L3*m2^2*m3*q2_p^2*sin(2*q2 + q3) - L1^2*L2*L3^3*m2*m3^2*q3_p^2*sin(2*q2 + q3) + 8*I2_zz*L1^2*L3^2*m3^2*q1_p*q2_p*sin(2*q2 + 2*q3) + 8*I2_zz*L1^2*L3^2*m3^2*q1_p*q3_p*sin(2*q2 + 2*q3) + 8*I2_zz*L1^2*L3^2*m3^2*q2_p*q3_p*sin(2*q2 + 2*q3) + 8*D1*L1*L2^2*L3*m3^2*q1_p*cos(q2 - q3) - 4*D1*L1*L2*L3^2*m3^2*q1_p*cos(q2 + 2*q3) - 8*D2*L1*L2^2*L3*m3^2*q2_p*cos(q2 - q3) + 4*D2*L1*L2*L3^2*m3^2*q2_p*cos(q2 + 2*q3) + 8*D2*L1^2*L2*L3*m3^2*q2_p*cos(2*q2 + q3) - 16*D3*L1^2*L2*L3*m3^2*q3_p*cos(2*q2 + q3) - 4*I3_zz*L1^3*L2*m1*m2*q1_p^2*sin(q2) - 8*I3_zz*L1^3*L2*m1*m3*q1_p^2*sin(q2) - 48*I3_zz*L1^3*L2*m2*m3*q1_p^2*sin(q2) + 4*I1_zz*L2^3*L3*m2*m3*q1_p^2*sin(q3) + 4*I1_zz*L2^3*L3*m2*m3*q2_p^2*sin(q3) + 8*I1_zz*L2*L3^3*m3^2*q1_p*q2_p*sin(q3) + 32*I1_zz*L2^3*L3*m3^2*q1_p*q2_p*sin(q3) + 8*I1_zz*L2*L3^3*m3^2*q1_p*q3_p*sin(q3) + 8*I1_zz*L2*L3^3*m3^2*q2_p*q3_p*sin(q3) + 16*D1*I3_zz*L1*L2*m2*q1_p*cos(q2) + 32*D1*I3_zz*L1*L2*m3*q1_p*cos(q2) - 16*D2*I3_zz*L1*L2*m2*q2_p*cos(q2) - 32*D2*I3_zz*L1*L2*m3*q2_p*cos(q2) - 16*D2*I1_zz*L2*L3*m3*q2_p*cos(q3) + 32*D3*I1_zz*L2*L3*m3*q3_p*cos(q3) + 8*I1_zz*L1*L2^2*L3*m3^2*q1_p^2*sin(q2 + q3) + 60*L1^2*L2*L3^2*g*m2*m3*cos(q1 - q2) + 10*L1^2*L2^2*L3*g*m1*m2*cos(q1 + q2 + q3) + 5*L1^2*L2^2*L3*g*m1*m3*cos(q1 + q2 + q3) + 15*L1^2*L2^2*L3*g*m2*m3*cos(q1 + q2 + q3) - 4*I1_zz*L1*L2*L3^2*m3^2*q1_p^2*sin(q2) + 8*I2_zz*L1^2*L2*L3*m3^2*q1_p^2*sin(q3) + 8*I2_zz*L1^2*L2*L3*m3^2*q2_p^2*sin(q3) + 8*I3_zz*L1^2*L2*L3*m3^2*q1_p^2*sin(q3) + 8*I3_zz*L1^2*L2*L3*m3^2*q2_p^2*sin(q3) + 8*I3_zz*L1^2*L2*L3*m3^2*q3_p^2*sin(q3) - 16*D3*L1^2*L2^2*m2*m3*q3_p*cos(2*q2) + 16*I1_zz*I2_zz*L1*L3*m3*q1_p^2*sin(q2 + q3) - 8*I1_zz*L1*L2^2*L3*m3^2*q1_p^2*sin(q2 - q3) + 4*I1_zz*L1*L2*L3^2*m3^2*q1_p^2*sin(q2 + 2*q3) + 8*I2_zz*L1^2*L2*L3*m3^2*q1_p^2*sin(2*q2 + q3) + 8*I2_zz*L1^2*L2*L3*m3^2*q2_p^2*sin(2*q2 + q3) - 8*I3_zz*L1^2*L2*L3*m3^2*q1_p^2*sin(2*q2 + q3) - 8*I3_zz*L1^2*L2*L3*m3^2*q2_p^2*sin(2*q2 + q3) - 8*I3_zz*L1^2*L2*L3*m3^2*q3_p^2*sin(2*q2 + q3) - 16*I1_zz*I3_zz*L1*L2*m2*q1_p^2*sin(q2) - 32*I1_zz*I3_zz*L1*L2*m3*q1_p^2*sin(q2) + 16*I1_zz*I2_zz*L2*L3*m3*q1_p^2*sin(q3) + 16*I1_zz*I2_zz*L2*L3*m3*q2_p^2*sin(q3) + 16*I1_zz*I3_zz*L2*L3*m3*q1_p^2*sin(q3) + 16*I1_zz*I3_zz*L2*L3*m3*q2_p^2*sin(q3) + 16*I1_zz*I3_zz*L2*L3*m3*q3_p^2*sin(q3) + 2*L1^2*L2^2*L3^2*m1*m3^2*q1_p^2*sin(2*q3) - 2*L1^2*L2^2*L3^2*m2*m3^2*q1_p^2*sin(2*q2) - L1^2*L2^2*L3^2*m2^2*m3*q1_p^2*sin(2*q2) + 2*L1^2*L2^2*L3^2*m1*m3^2*q2_p^2*sin(2*q3) + 4*L1^2*L2^2*L3^2*m2*m3^2*q1_p^2*sin(2*q3) - 2*L1^2*L2^2*L3^2*m2*m3^2*q2_p^2*sin(2*q2) - L1^2*L2^2*L3^2*m2^2*m3*q2_p^2*sin(2*q2) + L1^2*L2^2*L3^2*m1*m3^2*q3_p^2*sin(2*q3) + 4*L1^2*L2^2*L3^2*m2*m3^2*q2_p^2*sin(2*q3) + 2*L1^2*L2^2*L3^2*m2*m3^2*q3_p^2*sin(2*q3) - 35*L1^2*L2^2*L3*g*m1*m3*cos(q1 + q2 - q3) + 10*L1^2*L2*L3^2*g*m1*m3*cos(q1 + q2 + 2*q3) - 35*L1^2*L2^2*L3*g*m2*m3*cos(q1 + q2 - q3) + 30*L1^2*L2^2*L3*g*m2*m3*cos(q1 - q2 + q3) + 30*L1^2*L2*L3^2*g*m2*m3*cos(q1 + q2 + 2*q3) - 5*L1^2*L2^2*L3*g*m2*m3*cos(q1 + 3*q2 + q3) + 2*L1^3*L2^2*L3*m1*m3^2*q1_p^2*sin(q2 + q3) - 2*L1^3*L2^2*L3*m2^2*m3*q1_p^2*sin(q2 + q3) - 4*L1*L2*L3^2*m2*m3*tau1*cos(q2) + 4*L1*L2*L3^2*m2*m3*tau2*cos(q2) + 4*L1^2*L2*L3*m1*m3*tau2*cos(q3) - 8*L1^2*L2*L3*m1*m3*tau3*cos(q3) + 12*L1^2*L2*L3*m2*m3*tau2*cos(q3) - 24*L1^2*L2*L3*m2*m3*tau3*cos(q3) - 8*D1*L1*L2^2*L3*m3^2*q1_p*cos(q2 + q3) + 8*D2*L1*L2^2*L3*m3^2*q2_p*cos(q2 + q3) - L1^2*L2^2*L3^2*m2*m3^2*q1_p^2*sin(2*q2 + 2*q3) - L1^2*L2^2*L3^2*m2*m3^2*q2_p^2*sin(2*q2 + 2*q3) - L1^2*L2^2*L3^2*m2*m3^2*q3_p^2*sin(2*q2 + 2*q3) - 25*L1^2*L2*L3^2*g*m1*m3*cos(q1 + q2) - 40*L1^2*L2*L3^2*g*m2*m3*cos(q1 + q2) - 16*I3_zz*L1^2*L2^2*m2*m3*q1_p^2*sin(2*q2) - 16*I3_zz*L1^2*L2^2*m2*m3*q2_p^2*sin(2*q2) - L1^3*L2*L3^2*m1*m3^2*q1_p^2*sin(q2) + L1^2*L2*L3^3*m1*m3^2*q1_p^2*sin(q3) + 4*L1^2*L2^3*L3*m1*m3^2*q1_p^2*sin(q3) - 6*L1^3*L2*L3^2*m2*m3^2*q1_p^2*sin(q2) - 4*L1^3*L2*L3^2*m2^2*m3*q1_p^2*sin(q2) + L1^2*L2*L3^3*m1*m3^2*q2_p^2*sin(q3) + 3*L1^2*L2*L3^3*m2*m3^2*q1_p^2*sin(q3) + 4*L1^2*L2^3*L3*m1*m3^2*q2_p^2*sin(q3) + 6*L1^2*L2^3*L3*m2*m3^2*q1_p^2*sin(q3) + L1^2*L2^3*L3*m2^2*m3*q1_p^2*sin(q3) + L1^2*L2*L3^3*m1*m3^2*q3_p^2*sin(q3) + 3*L1^2*L2*L3^3*m2*m3^2*q2_p^2*sin(q3) + 6*L1^2*L2^3*L3*m2*m3^2*q2_p^2*sin(q3) + L1^2*L2^3*L3*m2^2*m3*q2_p^2*sin(q3) + 3*L1^2*L2*L3^3*m2*m3^2*q3_p^2*sin(q3) - 8*I3_zz*L1^2*L2^2*m2^2*q1_p*q2_p*sin(2*q2) - 32*I3_zz*L1^2*L2^2*m3^2*q1_p*q2_p*sin(2*q2) + 16*I1_zz*L2^2*L3^2*m3^2*q1_p*q2_p*sin(2*q3) + 8*I1_zz*L2^2*L3^2*m3^2*q1_p*q3_p*sin(2*q3) + 8*I1_zz*L2^2*L3^2*m3^2*q2_p*q3_p*sin(2*q3) - 4*L1*L2^2*L3*m2*m3*tau1*cos(q2 - q3) + 4*L1*L2^2*L3*m2*m3*tau2*cos(q2 - q3) - 4*L1^2*L2*L3*m2*m3*tau2*cos(2*q2 + q3) + 8*L1^2*L2*L3*m2*m3*tau3*cos(2*q2 + q3) + 4*D1*L1*L2*L3^2*m3^2*q1_p*cos(q2) - 4*D2*L1*L2*L3^2*m3^2*q2_p*cos(q2) - 8*D2*L1^2*L2*L3*m3^2*q2_p*cos(q3) + 16*D3*L1^2*L2*L3*m3^2*q3_p*cos(q3) + 4*I2_zz*L1^3*L3*m1*m3*q1_p^2*sin(q2 + q3) + 16*I2_zz*L1^3*L3*m2*m3*q1_p^2*sin(q2 + q3) + 2*L1^2*L2*L3^3*m1*m3^2*q1_p*q2_p*sin(q3) + 8*L1^2*L2^3*L3*m1*m3^2*q1_p*q2_p*sin(q3) + 2*L1^2*L2*L3^3*m1*m3^2*q1_p*q3_p*sin(q3) + 6*L1^2*L2*L3^3*m2*m3^2*q1_p*q2_p*sin(q3) + 12*L1^2*L2^3*L3*m2*m3^2*q1_p*q2_p*sin(q3) + 2*L1^2*L2^3*L3*m2^2*m3*q1_p*q2_p*sin(q3) + 2*L1^2*L2*L3^3*m1*m3^2*q2_p*q3_p*sin(q3) + 6*L1^2*L2*L3^3*m2*m3^2*q1_p*q3_p*sin(q3) + 6*L1^2*L2*L3^3*m2*m3^2*q2_p*q3_p*sin(q3) + 4*D1*L1*L2*L3^2*m2*m3*q1_p*cos(q2) - 4*D2*L1*L2*L3^2*m2*m3*q2_p*cos(q2) - 4*D2*L1^2*L2*L3*m1*m3*q2_p*cos(q3) - 12*D2*L1^2*L2*L3*m2*m3*q2_p*cos(q3) + 8*D3*L1^2*L2*L3*m1*m3*q3_p*cos(q3) + 24*D3*L1^2*L2*L3*m2*m3*q3_p*cos(q3) - L1^3*L2^2*L3*m1*m2*m3*q1_p^2*sin(q2 - q3) - 2*L1^2*L2*L3^3*m2*m3^2*q1_p*q2_p*sin(2*q2 + q3) - 4*L1^2*L2^3*L3*m2*m3^2*q1_p*q2_p*sin(2*q2 + q3) - 2*L1^2*L2^3*L3*m2^2*m3*q1_p*q2_p*sin(2*q2 + q3) - 2*L1^2*L2*L3^3*m2*m3^2*q1_p*q3_p*sin(2*q2 + q3) - 2*L1^2*L2*L3^3*m2*m3^2*q2_p*q3_p*sin(2*q2 + q3) + 4*D1*L1*L2^2*L3*m2*m3*q1_p*cos(q2 - q3) - 4*D2*L1*L2^2*L3*m2*m3*q2_p*cos(q2 - q3) + 4*D2*L1^2*L2*L3*m2*m3*q2_p*cos(2*q2 + q3) - 8*D3*L1^2*L2*L3*m2*m3*q3_p*cos(2*q2 + q3) + 8*I1_zz*L2^3*L3*m2*m3*q1_p*q2_p*sin(q3) - 4*I1_zz*L1*L2*L3^2*m2*m3*q1_p^2*sin(q2) + 4*I2_zz*L1^2*L2*L3*m1*m3*q1_p^2*sin(q3) + 4*I2_zz*L1^2*L2*L3*m1*m3*q2_p^2*sin(q3) + 12*I2_zz*L1^2*L2*L3*m2*m3*q1_p^2*sin(q3) + 4*I3_zz*L1^2*L2*L3*m1*m3*q1_p^2*sin(q3) + 12*I2_zz*L1^2*L2*L3*m2*m3*q2_p^2*sin(q3) + 4*I3_zz*L1^2*L2*L3*m1*m3*q2_p^2*sin(q3) + 12*I3_zz*L1^2*L2*L3*m2*m3*q1_p^2*sin(q3) + 4*I3_zz*L1^2*L2*L3*m1*m3*q3_p^2*sin(q3) + 12*I3_zz*L1^2*L2*L3*m2*m3*q2_p^2*sin(q3) + 12*I3_zz*L1^2*L2*L3*m2*m3*q3_p^2*sin(q3) + 16*I2_zz*L1^2*L2*L3*m3^2*q1_p*q2_p*sin(q3) + 16*I3_zz*L1^2*L2*L3*m3^2*q1_p*q2_p*sin(q3) + 16*I3_zz*L1^2*L2*L3*m3^2*q1_p*q3_p*sin(q3) + 16*I3_zz*L1^2*L2*L3*m3^2*q2_p*q3_p*sin(q3) - 4*I1_zz*L1*L2^2*L3*m2*m3*q1_p^2*sin(q2 - q3) + 4*I2_zz*L1^2*L2*L3*m2*m3*q1_p^2*sin(2*q2 + q3) + 4*I2_zz*L1^2*L2*L3*m2*m3*q2_p^2*sin(2*q2 + q3) - 4*I3_zz*L1^2*L2*L3*m2*m3*q1_p^2*sin(2*q2 + q3) - 4*I3_zz*L1^2*L2*L3*m2*m3*q2_p^2*sin(2*q2 + q3) - 4*I3_zz*L1^2*L2*L3*m2*m3*q3_p^2*sin(2*q2 + q3) + 16*I2_zz*L1^2*L2*L3*m3^2*q1_p*q2_p*sin(2*q2 + q3) - 16*I3_zz*L1^2*L2*L3*m3^2*q1_p*q2_p*sin(2*q2 + q3) - 16*I3_zz*L1^2*L2*L3*m3^2*q1_p*q3_p*sin(2*q2 + q3) - 16*I3_zz*L1^2*L2*L3*m3^2*q2_p*q3_p*sin(2*q2 + q3) + 32*I1_zz*I2_zz*L2*L3*m3*q1_p*q2_p*sin(q3) + 32*I1_zz*I3_zz*L2*L3*m3*q1_p*q2_p*sin(q3) + 32*I1_zz*I3_zz*L2*L3*m3*q1_p*q3_p*sin(q3) + 32*I1_zz*I3_zz*L2*L3*m3*q2_p*q3_p*sin(q3) + 4*L1^2*L2^2*L3^2*m1*m3^2*q1_p*q2_p*sin(2*q3) - 4*L1^2*L2^2*L3^2*m2*m3^2*q1_p*q2_p*sin(2*q2) - 2*L1^2*L2^2*L3^2*m2^2*m3*q1_p*q2_p*sin(2*q2) + 2*L1^2*L2^2*L3^2*m1*m3^2*q1_p*q3_p*sin(2*q3) + 8*L1^2*L2^2*L3^2*m2*m3^2*q1_p*q2_p*sin(2*q3) + 2*L1^2*L2^2*L3^2*m1*m3^2*q2_p*q3_p*sin(2*q3) + 4*L1^2*L2^2*L3^2*m2*m3^2*q1_p*q3_p*sin(2*q3) + 4*L1^2*L2^2*L3^2*m2*m3^2*q2_p*q3_p*sin(2*q3) - 2*L1^2*L2^2*L3^2*m2*m3^2*q1_p*q2_p*sin(2*q2 + 2*q3) - 2*L1^2*L2^2*L3^2*m2*m3^2*q1_p*q3_p*sin(2*q2 + 2*q3) - 2*L1^2*L2^2*L3^2*m2*m3^2*q2_p*q3_p*sin(2*q2 + 2*q3) - L1^3*L2*L3^2*m1*m2*m3*q1_p^2*sin(q2) + L1^2*L2^3*L3*m1*m2*m3*q1_p^2*sin(q3) + L1^2*L2^3*L3*m1*m2*m3*q2_p^2*sin(q3) - 32*I3_zz*L1^2*L2^2*m2*m3*q1_p*q2_p*sin(2*q2) + 2*L1^2*L2^3*L3*m1*m2*m3*q1_p*q2_p*sin(q3) + 8*I2_zz*L1^2*L2*L3*m1*m3*q1_p*q2_p*sin(q3) + 24*I2_zz*L1^2*L2*L3*m2*m3*q1_p*q2_p*sin(q3) + 8*I3_zz*L1^2*L2*L3*m1*m3*q1_p*q2_p*sin(q3) + 8*I3_zz*L1^2*L2*L3*m1*m3*q1_p*q3_p*sin(q3) + 24*I3_zz*L1^2*L2*L3*m2*m3*q1_p*q2_p*sin(q3) + 8*I3_zz*L1^2*L2*L3*m1*m3*q2_p*q3_p*sin(q3) + 24*I3_zz*L1^2*L2*L3*m2*m3*q1_p*q3_p*sin(q3) + 24*I3_zz*L1^2*L2*L3*m2*m3*q2_p*q3_p*sin(q3) + 8*I2_zz*L1^2*L2*L3*m2*m3*q1_p*q2_p*sin(2*q2 + q3) - 8*I3_zz*L1^2*L2*L3*m2*m3*q1_p*q2_p*sin(2*q2 + q3) - 8*I3_zz*L1^2*L2*L3*m2*m3*q1_p*q3_p*sin(2*q2 + q3) - 8*I3_zz*L1^2*L2*L3*m2*m3*q2_p*q3_p*sin(2*q2 + q3)))/(64*I1_zz*I2_zz*I3_zz + 16*I2_zz*I3_zz*L1^2*m1 + 16*I1_zz*I3_zz*L2^2*m2 + 64*I2_zz*I3_zz*L1^2*m2 + 16*I1_zz*I2_zz*L3^2*m3 + 64*I1_zz*I3_zz*L2^2*m3 + 64*I2_zz*I3_zz*L1^2*m3 + 8*I3_zz*L1^2*L2^2*m2^2 + 8*I1_zz*L2^2*L3^2*m3^2 + 8*I2_zz*L1^2*L3^2*m3^2 + 32*I3_zz*L1^2*L2^2*m3^2 - 8*I2_zz*L1^2*L3^2*m3^2*cos(2*q2 + 2*q3) + 2*L1^2*L2^2*L3^2*m1*m3^2 + 6*L1^2*L2^2*L3^2*m2*m3^2 + 2*L1^2*L2^2*L3^2*m2^2*m3 + 4*I3_zz*L1^2*L2^2*m1*m2 + 4*I2_zz*L1^2*L3^2*m1*m3 + 16*I3_zz*L1^2*L2^2*m1*m3 + 4*I1_zz*L2^2*L3^2*m2*m3 + 16*I2_zz*L1^2*L3^2*m2*m3 + 48*I3_zz*L1^2*L2^2*m2*m3 - 8*I3_zz*L1^2*L2^2*m2^2*cos(2*q2) - 32*I3_zz*L1^2*L2^2*m3^2*cos(2*q2) - 8*I1_zz*L2^2*L3^2*m3^2*cos(2*q3) - 32*I3_zz*L1^2*L2^2*m2*m3*cos(2*q2) + L1^2*L2^2*L3^2*m1*m2*m3 - 2*L1^2*L2^2*L3^2*m1*m3^2*cos(2*q3) - 4*L1^2*L2^2*L3^2*m2*m3^2*cos(2*q2) - 2*L1^2*L2^2*L3^2*m2^2*m3*cos(2*q2) - 4*L1^2*L2^2*L3^2*m2*m3^2*cos(2*q3) + 2*L1^2*L2^2*L3^2*m2*m3^2*cos(2*q2 + 2*q3));
    tau1_act = D1*q1_p + q3_pp*(I3_zz + (L3^2*m3)/4 + (L1*L3*m3*cos(q2 + q3))/2 + (L2*L3*m3*cos(q3))/2) + q1_pp*(I1_zz + I2_zz + I3_zz + (L1^2*m1)/4 + L1^2*m2 + L1^2*m3 + (L2^2*m2)/4 + L2^2*m3 + (L3^2*m3)/4 + L1*L3*m3*cos(q2 + q3) + L1*L2*m2*cos(q2) + 2*L1*L2*m3*cos(q2) + L2*L3*m3*cos(q3)) + (5*g*(7*L2*cos(q1 + q2) + 14*L1*cos(q1) + 2*L3*cos(q1 + q2 + q3)))/2 + q2_pp*(I2_zz + I3_zz + (L2^2*m2)/4 + L2^2*m3 + (L3^2*m3)/4 + (L1*L3*m3*cos(q2 + q3))/2 + (L1*L2*m2*cos(q2))/2 + L1*L2*m3*cos(q2) + L2*L3*m3*cos(q3)) - (L1*q2_p^2*(L3*m3*sin(q2 + q3) + L2*m2*sin(q2) + 2*L2*m3*sin(q2)))/2 - (L3*m3*q3_p^2*(L1*sin(q2 + q3) + L2*sin(q3)))/2 - L1*q1_p*q2_p*(L3*m3*sin(q2 + q3) + L2*m2*sin(q2) + 2*L2*m3*sin(q2)) - L3*m3*q1_p*q3_p*(L1*sin(q2 + q3) + L2*sin(q3)) - L3*m3*q2_p*q3_p*(L1*sin(q2 + q3) + L2*sin(q3));
    tau2_act = D2*q2_p + I2_zz*q1_pp + I2_zz*q2_pp + I3_zz*q1_pp + I3_zz*q2_pp + I3_zz*q3_pp + 5*L3*g*cos(q1 + q2 + q3) + (35*L2*g*cos(q1 + q2))/2 + (L2^2*m2*q1_pp)/4 + (L2^2*m2*q2_pp)/4 + L2^2*m3*q1_pp + L2^2*m3*q2_pp + (L3^2*m3*q1_pp)/4 + (L3^2*m3*q2_pp)/4 + (L3^2*m3*q3_pp)/4 + (L1*L2*m2*q1_p^2*sin(q2))/2 + L1*L2*m3*q1_p^2*sin(q2) - (L2*L3*m3*q3_p^2*sin(q3))/2 + (L1*L3*m3*q1_pp*cos(q2 + q3))/2 + (L1*L2*m2*q1_pp*cos(q2))/2 + L1*L2*m3*q1_pp*cos(q2) + L2*L3*m3*q1_pp*cos(q3) + L2*L3*m3*q2_pp*cos(q3) + (L2*L3*m3*q3_pp*cos(q3))/2 + (L1*L3*m3*q1_p^2*sin(q2 + q3))/2 - L2*L3*m3*q1_p*q3_p*sin(q3) - L2*L3*m3*q2_p*q3_p*sin(q3);
    tau3_act = (L3*m3*(L1*sin(q2 + q3) + L2*sin(q3))*q1_p^2)/2 + L2*L3*m3*sin(q3)*q1_p*q2_p + (L2*L3*m3*sin(q3)*q2_p^2)/2 + D3*q3_p + q2_pp*((m3*L3^2)/4 + (L2*m3*cos(q3)*L3)/2 + I3_zz) + q1_pp*(I3_zz + (L3^2*m3)/4 + (L1*L3*m3*cos(q2 + q3))/2 + (L2*L3*m3*cos(q3))/2) + q3_pp*((m3*L3^2)/4 + I3_zz) + 5*L3*g*cos(q1 + q2 + q3);
    output = [q1_p, q2_p, q3_p, q1_pp, q2_pp, q3_pp, tau1_act, tau2_act, tau3_act];
end

== matlab function rmc_simulation/get tau ==
  data: input input; output output
function output  = get_tau(input)
    tau1 = input(7);
    tau2 = input(8);
    tau3 = input(9);
    output = [tau1, tau2, tau3];
end

== matlab function rmc_simulation/saturate pi ==
  data: input input; output output
function output  = saturate_pi(input)
    q1 = input(1);
    q2 = input(2);
    q3 = input(3);
    q1_p = input(4);
    q2_p = input(5);
    q3_p = input(6); 
    q1 = atan2(sin(q1),cos(q1));
    q2 = atan2(sin(q2),cos(q2));
    q3 = atan2(sin(q3),cos(q3));
    output = [q1, q2, q3, q1_p, q2_p, q3_p];
end

== matlab function rmc_simulation/get q ==
  data: input input; q1_p output; q2_p output; q3_p output; q1_pp output; q2_pp output; q3_pp output
function [q1_p, q2_p, q3_p, q1_pp, q2_pp, q3_pp]  = get_q(input)
    q1_p = input(1);
    q2_p = input(2);
    q3_p = input(3);
    q1_pp = input(4);
    q2_pp = input(5);
    q3_pp = input(6);
    %output = [q1_p, q2_p, q3_p, q1_pp, q2_pp, q3_pp];
end

== matlab function rmc_simulation/tau solve ==
  data: input input; output output
function output  = tau_solve(input)
    q1_pp = input(1);
    q2_pp = input(2);
    q3_pp = input(3);
    L1 = input(4);
    L2 = input(5);
    L3 = input(6);
    m1 = input(7);
    m2 = input(8);
    m3 = input(9);
    I1_zz = input(10);
    I2_zz = input(11);
    I3_zz = input(12);
    g = input(13);
    D1 = input(14);
    D2 = input(15);
    D3 = input(16);
    q1 = input(17);
    q2 = input(18);
    q3 = input(19);
    q1_p = input(20);
    q2_p = input(21);
    q3_p = input(22);
    q1 = q1 - 2*pi*floor((q1+pi)/(2*pi));
    q2 = q2 - 2*pi*floor((q2+pi)/(2*pi));
    q3 = q3 - 2*pi*floor((q3+pi)/(2*pi));
%     q1 = atan2(sin(q1),cos(q1));
%     q2 = atan2(sin(q2),cos(q2));
%     q3 = atan2(sin(q3),cos(q3));
    tau1_des = D1*q1_p + q3_pp*(I3_zz + (L3^2*m3)/4 + (L1*L3*m3*cos(q2 + q3))/2 + (L2*L3*m3*cos(q3))/2) + q1_pp*(I1_zz + I2_zz + I3_zz + (L1^2*m1)/4 + L1^2*m2 + L1^2*m3 + (L2^2*m2)/4 + L2^2*m3 + (L3^2*m3)/4 + L1*L3*m3*cos(q2 + q3) + L1*L2*m2*cos(q2) + 2*L1*L2*m3*cos(q2) + L2*L3*m3*cos(q3)) + (5*g*(7*L2*cos(q1 + q2) + 14*L1*cos(q1) + 2*L3*cos(q1 + q2 + q3)))/2 + q2_pp*(I2_zz + I3_zz + (L2^2*m2)/4 + L2^2*m3 + (L3^2*m3)/4 + (L1*L3*m3*cos(q2 + q3))/2 + (L1*L2*m2*cos(q2))/2 + L1*L2*m3*cos(q2) + L2*L3*m3*cos(q3)) - (L1*q2_p^2*(L3*m3*sin(q2 + q3) + L2*m2*sin(q2) + 2*L2*m3*sin(q2)))/2 - (L3*m3*q3_p^2*(L1*sin(q2 + q3) + L2*sin(q3)))/2 - L1*q1_p*q2_p*(L3*m3*sin(q2 + q3) + L2*m2*sin(q2) + 2*L2*m3*sin(q2)) - L3*m3*q1_p*q3_p*(L1*sin(q2 + q3) + L2*sin(q3)) - L3*m3*q2_p*q3_p*(L1*sin(q2 + q3) + L2*sin(q3));
    tau2_des = D2*q2_p + I2_zz*q1_pp + I2_zz*q2_pp + I3_zz*q1_pp + I3_zz*q2_pp + I3_zz*q3_pp + 5*L3*g*cos(q1 + q2 + q3) + (35*L2*g*cos(q1 + q2))/2 + (L2^2*m2*q1_pp)/4 + (L2^2*m2*q2_pp)/4 + L2^2*m3*q1_pp + L2^2*m3*q2_pp + (L3^2*m3*q1_pp)/4 + (L3^2*m3*q2_pp)/4 + (L3^2*m3*q3_pp)/4 + (L1*L2*m2*q1_p^2*sin(q2))/2 + L1*L2*m3*q1_p^2*sin(q2) - (L2*L3*m3*q3_p^2*sin(q3))/2 + (L1*L3*m3*q1_pp*cos(q2 + q3))/2 + (L1*L2*m2*q1_pp*cos(q2))/2 + L1*L2*m3*q1_pp*cos(q2) + L2*L3*m3*q1_pp*cos(q3) + L2*L3*m3*q2_pp*cos(q3) + (L2*L3*m3*q3_pp*cos(q3))/2 + (L1*L3*m3*q1_p^2*sin(q2 + q3))/2 - L2*L3*m3*q1_p*q3_p*sin(q3) - L2*L3*m3*q2_p*q3_p*sin(q3);
    tau3_des = (L3*m3*(L1*sin(q2 + q3) + L2*sin(q3))*q1_p^2)/2 + L2*L3*m3*sin(q3)*q1_p*q2_p + (L2*L3*m3*sin(q3)*q2_p^2)/2 + D3*q3_p + q2_pp*((m3*L3^2)/4 + (L2*m3*cos(q3)*L3)/2 + I3_zz) + q1_pp*(I3_zz + (L3^2*m3)/4 + (L1*L3*m3*cos(q2 + q3))/2 + (L2*L3*m3*cos(q3))/2) + q3_pp*((m3*L3^2)/4 + I3_zz) + 5*L3*g*cos(q1 + q2 + q3);
    output = [tau1_des, tau2_des, tau3_des];
end
